simulink model "heat_exchange_bypass_logic"  (R2020b)
settings: Solver=VariableStepAuto  StartTime=0.0  StopTime=10.0  RelTol=1e-3
settings Model: Creator=Litao  LastModifiedBy=Litao

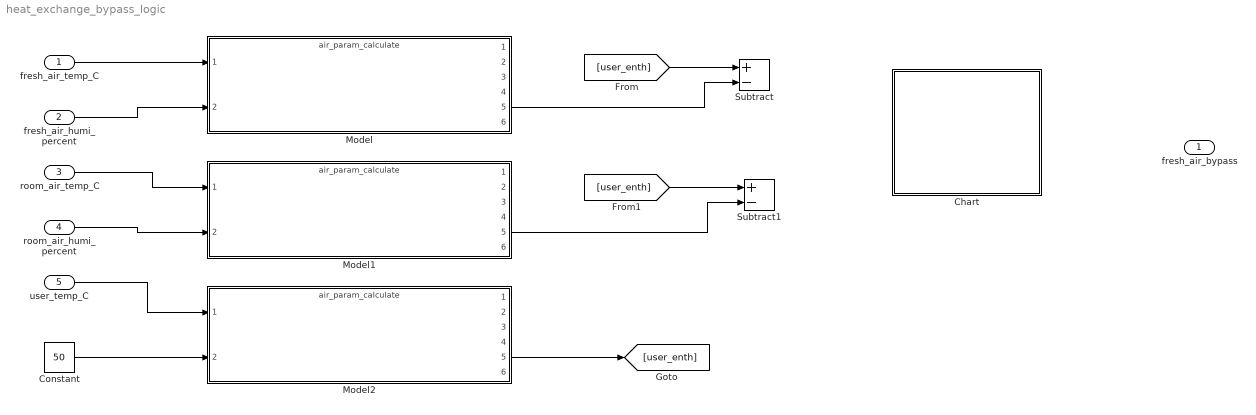
== system heat_exchange_bypass_logic ==
  fresh_air_temp_C : Inport
  fresh_air_humi_percent : Inport  Port=2
  room_air_temp_C : Inport  Port=3
  room_air_humi_percent : Inport  Port=4
  user_temp_C : Inport  Port=5
  Chart : Stateflow chart  TreatAsAtomicUnit=on
  Constant : Constant  Value=50
  Model : ModelReference  ModelNameDialog=air_param_calculate.slx  SimulationMode=Normal  ModelReferenceVersion=1.16
  Model1 : ModelReference  ModelNameDialog=air_param_calculate.slx  SimulationMode=Normal  ModelReferenceVersion=1.16
  Model2 : ModelReference  ModelNameDialog=air_param_calculate.slx  SimulationMode=Normal  ModelReferenceVersion=1.16
  Subtract : Sum  Inputs=+-
  Subtract1 : Sum  Inputs=+-
  fresh_air_bypass : Outport
  wires:
  fresh_air_temp_C/1 -> Model/1
  fresh_air_humi_percent/1 -> Model/2
  room_air_temp_C/1 -> Model1/1
  room_air_humi_percent/1 -> Model1/2
  user_temp_C/1 -> Model2/1
  Constant/1 -> Model2/2
  Model2/5 -> [user_enth]
  [user_enth] -> Subtract/1
  Model/5 -> Subtract/2
  [user_enth] -> Subtract1/1
  Model1/5 -> Subtract1/2

== stateflow chart heat_exchange_bypass_logic/Chart ==
